simulink model "rtwdemo_sil_modelblock"  (Simulink 7.6)
settings: Solver=FixedStepDiscrete  SolverMode=SingleTasking  StartTime=0.0  StopTime=10  FixedStep=T  RelTol=1e-3
PostLoadFcn:
  | rtwdemo_overrides='{''LaunchReport'',''PassReuseOutputArgsAs''}';
  | rtwconfiguredemo(gcs,'noop',false,rtwdemo_overrides);
  | rtwdemo_cs=getActiveConfigSet(gcs);
  | setProp(rtwdemo_cs,'CustomSymbolStr','$R$N$M');
  | set_param(gcs,'dirty','off');
  | clear rtwdemo_overrides rtwdemo_cs
  | 
  | rtwdemo_sil_modelblock_data
undefined symbols (not defined in the file or in its folder): myLower, myUpper, T
Description:
  | Processor-in-the-Loop Code Verification
CloseFcn:
  | try, close_system('rtwdemo_pil2_counter',0), end
settings Model: Creator=The MathWorks Inc.  ExtModeAutoUpdateStatusClock=off
settings MATStruct: SampleTime=0.1  Offset=0  Priority=[20.0]
settings DataIOCC: LimitDataPoints=off  SaveFormat=StructureWithTime  SaveOutput=off  SaveTime=off  ReturnWorkspaceOutputs=on  SignalLoggingName=logsOut
settings OptimizationCC: InlineParams=on  UseIntDivNetSlope=on  InlineInvariantSignals=on  EnhancedBackFolding=on  BooleansAsBitfields=on  PassReuseOutputArgsAs=Individual arguments  StateBitsets=on  DataBitsets=on  UseTempVars=on  ZeroExternalMemoryAtStartup=off  ZeroInternalMemoryAtStartup=off  NoFixptDivByZeroProtection=on  EfficientFloat2IntCast=on  OptimizeModelRefInitCode=on  LifeSpan=1  SimCompilerOptimization=On
settings DebuggingCC: MergeDetectMultiDrivingBlocksExec=error  CheckExecutionContextPreStartOutputMsg=on  CheckExecutionContextRuntimeOutputMsg=on  SolverPrmCheckMsg=none  UniqueDataStoreMsg=error  ModelReferenceSymbolNameMessage=none  StrictBusMsg=ErrorOnBusTreatedAsVector
settings HardwareCC: ProdIntDivRoundTo=Zero  ProdEndianess=LittleEndian  ProdHWDeviceType=Specified  TargetHWDeviceType=Generic->32-bit Embedded Processor
settings ModelReferenceCC: CheckModelReferenceTargetMessage=none
settings RTWCC: SystemTargetFile=ert.tlc  TLCOptions=-p0 -aWarnNonSaturatedBlocks=0  TemplateMakefile=ert_default_tmf  Description=Real-Time Workshop Embedded Coder  GenerateReport=on  RTWVerbose=off  ProcessScript=ert_make_rtw_hook  IncludeHyperlinkInReport=on  GenerateTraceInfo=on  GenerateTraceReport=on  GenerateTraceReportSl=on  GenerateTraceReportSf=on  GenerateTraceReportEml=on
settings CodeAppCC: ForceParamTrailComments=on  IgnoreCustomStorageClasses=off  IgnoreTestpoints=on  SimulinkDataObjDesc=on  CustomSymbolStrGlobalVar=rt$N$M  CustomSymbolStrType=$N$M  CustomSymbolStrFcn=$N$M$F  CustomSymbolStrMacro=$N$M  InsertBlockDesc=on
settings ERTTargetCC: MultiwordLength=2048  GenerateSampleERTMain=on  IncludeMdlTerminateFcn=off  CombineSignalStateStructs=on  SupportNonFinite=off  SupportComplex=off  InlinedParameterPlacement=NonHierarchical  ERTCustomFileTemplate=example_file_process.tlc  ERTFilePackagingFormat=CompactWithDataFile  ConvertIfToSwitch=off

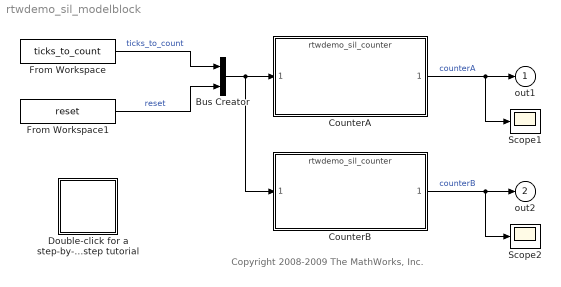
== system rtwdemo_sil_modelblock ==
  note: Copyright 2008-2009 The MathWorks, Inc.
  Bus Creator : BusCreator  Inputs='ticks_to_count','reset'  OutDataTypeStr=Bus: SilCounterBus  NonVirtualBus=on
  CounterA : ModelReference  ModelNameDialog=rtwdemo_sil_counter  ParameterArgumentNames=myLower,myUpper  ParameterArgumentValues=40 70  SimulationMode=Software-in-the-loop (SIL)  ModelReferenceVersion=1.123  CopyOfModelName=rtwdemo_sil_counter
  CounterB : ModelReference  ModelNameDialog=rtwdemo_sil_counter  ParameterArgumentNames=myLower,myUpper  ParameterArgumentValues=40 70  SimulationMode=Normal  ModelReferenceVersion=1.123  CopyOfModelName=rtwdemo_sil_counter
  Double-click for a step-by-step tutorial : Subsystem
      settings: OpenFcn=showdemo('rtwdemo_sil_pil_script');
      mask Type: Info
      mask Display: image(imread('targets_demo_info.bmp','bmp'),'center')
  From Workspace : FromWorkspace  VariableName=ticks_to_count  SampleTime=T
  From Workspace1 : FromWorkspace  VariableName=reset  SampleTime=T
  Scope1 : Scope
      settings: TimeRange=10  YMin=0  YMax=100
  Scope2 : Scope
      settings: TimeRange=10  YMin=0  YMax=100
  out1 : Outport
  out2 : Outport  Port=2
  wires:
  CounterA/1 -> Scope1/1, out1/1  "counterA"
  Bus Creator/1 -> CounterA/1, CounterB/1
  From Workspace/1 -> Bus Creator/1  "ticks_to_count"
  From Workspace1/1 -> Bus Creator/2  "reset"
  CounterB/1 -> out2/1, Scope2/1  "counterB"

== system rtwdemo_sil_modelblock/Double-click for a step-by-step tutorial ==
